simulink model "IO601candatabaseloopback"  (R2013b)
settings: Solver=FixedStepDiscrete  StartTime=0.0  StopTime=inf  RelTol=1e-3
libraries: speedgoatlib_IO601 x3, canmsglib x2, xpclib x1
Description:
  | 7.14.0.739 (R2012a)
settings Model: BufferReuse=off  Creator=cedric  LastModifiedBy=lab3
settings SolverCC: EnableConcurrentExecution=on
settings DataIOCC: SignalLoggingSaveFormat=ModelDataLogs
settings OptimizationCC: BlockReduction=off  OptimizeBlockIOStorage=off  BufferReuse=off  ExpressionFolding=off  ExpressionDepthLimit=2147483647  LocalBlockOutputs=off
settings DebuggingCC: FcnCallInpInsideContextMsg=UseLocalSettings  StateNameClashWarn=warning
settings HardwareCC: ProdIntDivRoundTo=Zero  ProdEndianess=LittleEndian  ProdHWDeviceType=Generic->32-bit x86 compatible
settings RTWCC: SystemTargetFile=xpctarget.tlc  TemplateMakefile=xpc_default_tmf  Description=Simulink Real-Time  RTWVerbose=off  ProcessScript=xpctarget_make_rtw_hook  RTWCompilerOptimization=On
settings xpcTargetCC: TargetFcnLib=ansi_tfl_table_tmw.mat  CodeReplacementLibrary=XPC_BLAS  ParMdlRefBuildCompliant=on  ConcurrentExecutionCompliant=on  CombineSignalStateStructs=off  MATLABClassNameForMDSCustomization=xpcAperiodicCustomization  GRTInterface=on  GenerateAllocFcn=off  xPCTaskExecutionProfile=off  xPCRL32EventNumber=5000  xPCLoadParamSetFile=off  xPCConcurrentTasks=off  xPCEnableSFAnimation=off

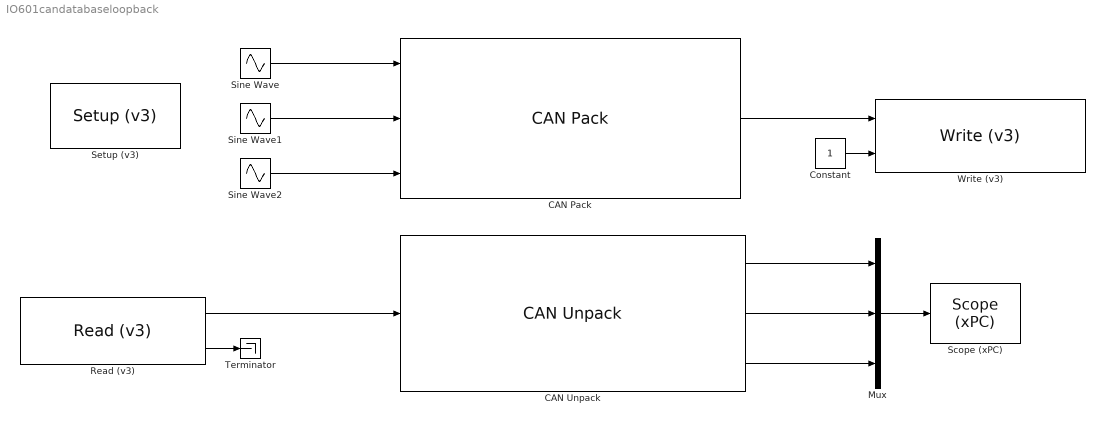
== system IO601candatabaseloopback ==
  CAN Pack : canmsglib/CAN Pack  CANdbFile=C:\Users\dkuratli\Documents\MATLAB\speedgoatlib_branch_8_test1\thirdpartydrivers\sg_help\examples\IO601candatabase_db.dbc  MsgList=TripDistance  MsgName=TripDistance  MsgIDType=Extended (29-bit identifier)  MsgIdentifier=486455808  MsgLength=8  SignalInfo=TripDistanceGearDown$0$16$1$2$1$0$1$0$0$65535$#TripDistanceTopGear$16$16$1$2$1$0$1$0$0$65535$#TripDistanceVSL$32$16$1$2$1$0$1$0$0$65535$#  NSignals=3  StartBits=str2num('[int32(0);int32(16);int32(32)]')  SignalSizes=str2num('[int32(16);int32(16);int32(16)]')  ByteOrders=str2num('[int32(1);int32(1);int32(1)]')  DataTypes=str2num('[int32(2);int32(2);int32(2)]')  MultiplexTypes=str2num('[int32(1);int32(1);int32(1)]')  MultiplexValues=str2num('[double(0);double(0);double(0)]')  Factors=str2num('[double(1);double(1);double(1)]')  Offsets=str2num('[double(0);double(0);double(0)]')  Minimums=str2num('[double(0);double(0);double(0)]')  Maximums=str2num('[double(65535);double(65535);double(65535)]')  Remote=off
      settings: DataFormat=CANdb specified signals
  CAN Unpack : canmsglib/CAN Unpack  CANdbFile=C:\Users\dkuratli\Documents\MATLAB\speedgoatlib_branch_8_test1\thirdpartydrivers\sg_help\examples\IO601candatabase_db.dbc  MsgList=TripDistance  MsgName=TripDistance  MsgIDType=Extended (29-bit identifier)  MsgIdentifier=486455808  MsgLength=8  SignalInfo=TripDistanceGearDown$0$16$1$2$1$0$1$0$0$65535$#TripDistanceTopGear$16$16$1$2$1$0$1$0$0$65535$#TripDistanceVSL$32$16$1$2$1$0$1$0$0$65535$#  NSignals=3  IDPort=off  TimestampPort=off  ErrorPort=off  RemotePort=off  LengthPort=off  StatusPort=off  StartBits=str2num('[int32(0);int32(16);int32(32)]')  SignalSizes=str2num('[int32(16);int32(16);int32(16)]')  ByteOrders=str2num('[int32(1);int32(1);int32(1)]')  DataTypes=str2num('[int32(2);int32(2);int32(2)]')  MultiplexTypes=str2num('[int32(1);int32(1);int32(1)]')  MultiplexValues=str2num('[double(0);double(0);double(0)]')  Factors=str2num('[double(1);double(1);double(1)]')  Offsets=str2num('[double(0);double(0);double(0)]')  Minimums=str2num('[double(0);double(0);double(0)]')  Maximums=str2num('[double(65535);double(65535);double(65535)]')
      settings: DataFormat=CANdb specified signals
  Constant : Constant
  Mux : Mux  Inputs=3
  Read (v3) : speedgoatlib_IO601/Read (v3)  id=1  outputFormat=Vector of CAN_MESSAGE  port1=off  port2=on  depth1=1  depth2=1  sampletime=0.001  pciSlot=-1
  "Scope (xPC) " : xpclib/Misc./Scope (xPC)   scopeno=1  scopetype=Target  autostart=on  viewmode=Graphical redraw  formatstr='%15.6f'  grid=on  ylimits=[0,0]  nosamples=390  noprepostsamples=0  interleave=1  triggermode=Signal triggering  triggersignal=1  trigsignalfromport=off  triggerlevel=1  triggerslope=Rising  triggerscope=1  triggersample=0  filename=data.dat  mode=Lazy  writesize=512  autorestart=off  dynamicfilemode=off  maxwritefilesize=512*1024^2
  Setup (v3) : speedgoatlib_IO601/Setup (v3)  id=1  can1enable=on  can1bus=Highspeed  can1Baudrate=1 MBaud  can1UserBR=[1,1,5,2]  stdAcc1=[0,0,0,0]  extAcc1=[0,0,0,0]  can2enable=on  can2bus=Highspeed  can2Baudrate=1 MBaud  can2UserBR=[1,1,5,2]  stdAcc2=[0,0,0,0]  extAcc2=[0,0,0,0]  pciSlot=-1
  Sine Wave : Sin  Amplitude=200  Bias=200  Frequency=2*pi*80
  Sine Wave1 : Sin  Amplitude=200  Bias=200  Frequency=2*pi*20  Phase=pi/2
  Sine Wave2 : Sin  Amplitude=200  Bias=200  Frequency=2*pi*2  Phase=pi
  Terminator : Terminator
  Write (v3) : speedgoatlib_IO601/Write (v3)  Priority=1  id=1  sampletime=0.001  pciSlot=-1  inputType=CAN_MESSAGE plus count  port=1  maxMsg=1  status=off  init=[]  term=[]
  wires:
  CAN Pack/1 -> Write (v3)/1
  Read (v3)/1 -> CAN Unpack/1
  Sine Wave/1 -> CAN Pack/1
  Mux/1 -> "Scope (xPC) "/1
  CAN Unpack/1 -> Mux/1
  CAN Unpack/2 -> Mux/2
  CAN Unpack/3 -> Mux/3
  Read (v3)/2 -> Terminator/1
  Constant/1 -> Write (v3)/2
  Sine Wave1/1 -> CAN Pack/2
  Sine Wave2/1 -> CAN Pack/3
